simulink library "speedgoatlib_IO723"  (R2024b)
settings: Solver=VariableStepAuto  StartTime=0.0  StopTime=10.0  RelTol=1e-3  EnableMultiTasking=on
undefined symbols (not defined in the file): sg_io723_manipulation_m, sg_io723_read_m, sg_io723_write_m, sgrestbus
settings Model: sg_rtwmakecfg_data=_a664api_  Creator=mrusconi  LastModifiedBy=speedgoat\jenkins
settings SolverCC: AlgebraicLoopSolver=TrustRegion
settings DataIOCC: LimitDataPoints=on  ReturnWorkspaceOutputs=off
settings OptimizationCC: ReuseModelBlockBuffer=off  LifeSpan=inf
settings DebuggingCC: UnconnectedInputMsg=warning  UnconnectedOutputMsg=warning  UnconnectedLineMsg=warning  AllowSymbolicDim=off  PregeneratedLibrarySubsystemCodeDiagnostic=none  SFUnexpectedBacktrackingDiag=warning  SFNoUnconditionalDefaultTransitionDiag=warning  SFExecutionAtInitializationDiag=none  ArithmeticOperatorsInVariantConditions=warning
settings ModelReferenceCC: EnableRefExpFcnMdlSchedulingChecks=on  PropagateSignalLabelsOutOfModel=off
settings SFSimCC: SimUseLocalCustomCode=off  CustomCodeUndefinedFunction=UseInterfaceOnly
settings RTWCC: RTWUseLocalCustomCode=off  GPUComputeCapability=3.5  DLArmComputeVersion=19.05
settings CodeAppCC: StateflowObjectComments=on
settings GRTTargetCC: TargetLangStandard=C89/C90 (ANSI)
settings ConfigComp: CovMetricSettings=dw  CovSaveCumulativeToWorkspaceVar=on  CovSaveSingleToWorkspaceVar=on  CovExternalEMLEnable=off  CovBoundaryAbsTol=1.0e-5

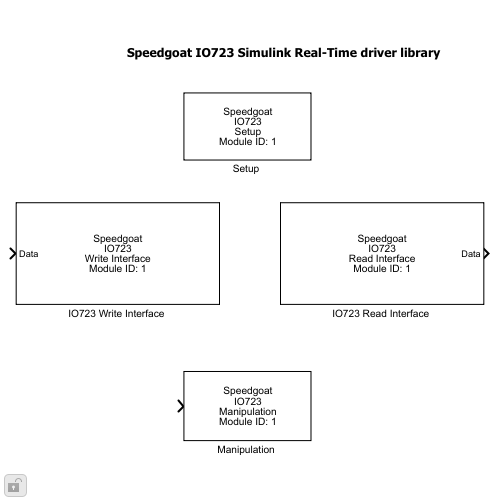
[thumbnail: Simulink's stored preview of the top-level diagram]
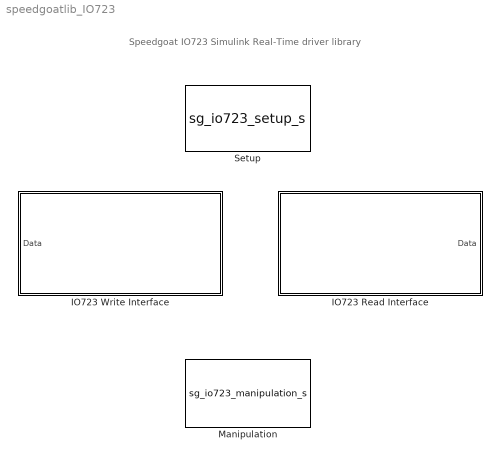
== system speedgoatlib_IO723 ==
  note: Speedgoat IO723 Simulink Real-Time driver library
  "IO723 Read Interface " : Subsystem  InitFcn=sgrestbus.checkRBSver(gcb);
      settings: CopyFcn=sgrestbus.gui.CopyFcnIO723Interface(gcb);  OpenFcn=sgrestbus.gui.OpenFcnIO723Interface();
      mask Help: eval('sg.utils.help.show(''io_main/refentry_io723_read_interface'');')
      mask Display: disp('Speedgoat\nIO723\nRead Interface\nModule ID: 1');
  "IO723 Write Interface " : Subsystem  InitFcn=sgrestbus.checkRBSver(gcb);
      settings: CopyFcn=sgrestbus.gui.CopyFcnIO723Interface(gcb);  OpenFcn=sgrestbus.gui.OpenFcnIO723Interface();
      mask Help: eval('sg.utils.help.show(''io_main/refentry_io723_write_interface'');')
      mask Display: disp('Speedgoat\nIO723\nWrite Interface\nModule ID: 1');
  "Manipulation " : S-Function  LoadFcn=sg_io723_manipulation_m.initBus();  InitFcn=sg_io723_manipulation_m.runInitFcn()  FunctionName=sg_io723_manipulation_s  Parameters=parModuleId, parSampleTime, parManipulations, parSequences, parEnValue  SFunctionDeploymentMode=off  EnableBusSupport=off  mask(manipulation_IO723){parModuleId=1, parSampleTime=-1, parEnValue=Database, parManipulations=0, parManipNames=0, parSequences=0}
      mask prompts: parModuleId "Module ID"; parSampleTime "Sample Time [s]"; parEnValue "Manipulation Value Source"; parManipulations "Manipulations"; parManipNames "Manipulation Names"; parSequences "Sequences"
      mask help: Speedgoat Driver Block<br>IO723 - Manipulation<br><br>&copy; 2007 - 2026, Speedgoat GmbH, <a href="matlab: web('www.speedgoat.com','-browser');">www.speedgoat.com</a>
      mask init:
      | sg_io723_manipulation_m.runMaskInit()
      settings: CopyFcn=sg_io723_manipulation_m.initBus();
      mask Help: eval('sg.utils.help.show(''io_main/refentry_io723_manipulation'');')
      mask TypeOptions parEnValue: Database | Block Input
      mask Callback parEnValue: sg_io723_manipulation_m.initBus();
      mask Display: disp('Speedgoat\nIO723\nManipulation\nModule ID: 1');
  "Setup " : S-Function  InitFcn=|  FunctionName=sg_io723_setup_s  Parameters=parModuleId, parPciSlot, parFPGAver, parRBSver  SFunctionModules=sg_IO723  SFunctionDeploymentMode=off  EnableBusSupport=off  mask(setup_IO723){parModuleId=1, parPciSlot=-1, parProject='', parFPGAver=[0,0], parRBSver=0}
      | sg.block.init();
      | sg_io723_setup_m.runInitFcn()
      mask prompts: parModuleId "Module ID"; parPciSlot "PCI Slot (-1: autosearch)"; parProject "Project File"; parFPGAver "FPGA Version/Type"; parRBSver "RBS Timestamp"
      mask help: Speedgoat Driver Block<br>IO723 - Setup<br><br>&copy; 2007 - 2024, Speedgoat GmbH, <a href="matlab: web('www.speedgoat.com','-browser');">www.speedgoat.com</a>
      mask init:
      | sg_io723_setup_m.runMaskInit()
      mask Help: eval('sg.utils.help.show(''io_main/refentry_ref_io723'');')
      mask Callback parProject: sg_io723_setup_m.projectFileClb()
      mask DialogControl Container4 Prompt: Module Settings
      mask DialogControl Container3 Prompt: Module Configuration
      mask DialogControl btnBrowse Prompt: Browse
      mask DialogControl btnBrowse Callback: sg_io723_setup_m.browseBtnClb()
      mask DialogControl btnUpdate Prompt: Update
      mask DialogControl btnUpdate Callback: sg_io723_setup_m.updateBtnClb();
      mask Display: disp('Speedgoat\nIO723\nSetup\nModule ID: 1');

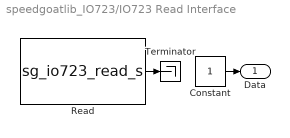
== system speedgoatlib_IO723/IO723 Read Interface  ==
  Constant : Constant  OutDataTypeStr=uint8
  "Read " : S-Function  InitFcn=sg_io723_write_m.runInitFcn()  FunctionName=sg_io723_read_s  Parameters=parModuleId, parPciSlot, parSampleTime, parSignalId, parSignalLen, parOutType  SFunctionDeploymentMode=off  EnableBusSupport=off  mask(read_IO723){parModuleId=1, parSignalId=0, parSignalLen=1, parOutType=1, parSampleTime=0.01, parPciSlot=-1}
      mask prompts: parModuleId "Module ID"; parSignalId "Signal ID"; parSignalLen "Signal Length"; parOutType "Output Data Type"; parSampleTime "Sample Time"; parPciSlot "PCI Slot (-1: autosearch)"
      mask help: Speedgoat Driver Block<br>IO723 - Read<br><br>&copy; 2007 - 2026, Speedgoat GmbH, <a href="matlab: web('www.speedgoat.com','-browser');">www.speedgoat.com</a>
      mask init:
      | sg_io723_read_m.runMaskInit()
      mask Help: eval('sg.utils.help.show(''io_main/refentry_ref_io723'');')
      mask Display: disp('Speedgoat\nIO723\nRead\nModule ID: 1');
  Terminator : Terminator
  Data : Outport
  wires:
  "Read "/1 -> Terminator/1
  Constant/1 -> Data/1

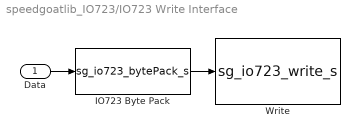
== system speedgoatlib_IO723/IO723 Write Interface  ==
  Data : Inport
  IO723 Byte Pack : S-Function  FunctionName=sg_io723_bytePack_s  Parameters=outWidth  SFunctionDeploymentMode=off  EnableBusSupport=off  mask{outWidth=1}
      mask prompts: outWidth "Output Port Size"
      mask help: Speedgoat Driver Block<br>IO723 - Byte Pack<br><br>This block converts the input data to a uint8 vector, which length is defined by the Output Port Size parameter. Byte padding or truncation is applied in case the size of the input data does not match the defined output size. <br><br>&copy; 2007 - 2024, Speedgoat GmbH, <a href="matlab: web('www.speedgoat.com','-browser');">www.speedgoat.com</a>
      mask Help: eval('sg.utils.help.show(''io_main/refentry_ref_io723'');')
      mask Display: disp('Speedgoat\nIO723\nByte Pack');
  "Write " : S-Function  InitFcn=sg_io723_read_m.runInitFcn()  FunctionName=sg_io723_write_s  Parameters=parModuleId, parPciSlot, parSampleTime, parSignalId, parSignalLen, parInpType  SFunctionDeploymentMode=off  EnableBusSupport=off  mask(write_IO723){parModuleId=1, parSignalId=0, parSignalLen=1, parInpType=1, parSampleTime=-1, parPciSlot=-1}
      mask prompts: parModuleId "Module ID"; parSignalId "Signal ID"; parSignalLen "Signal Length"; parInpType "Input Data Type"; parSampleTime "Sample Time"; parPciSlot "PCI Slot (-1: autosearch)"
      mask help: Speedgoat Driver Block<br>IO723 - Write<br><br>&copy; 2007 - 2026, Speedgoat GmbH, <a href="matlab: web('www.speedgoat.com','-browser');">www.speedgoat.com</a>
      mask init:
      | sg_io723_write_m.runMaskInit();
      mask Help: eval('sg.utils.help.show(''io_main/refentry_ref_io723'');')
      mask Display: disp('Speedgoat\nIO723\nWrite\nModule ID: 1');
  wires:
  Data/1 -> IO723 Byte Pack/1
  IO723 Byte Pack/1 -> "Write "/1
